simulink model "pendulumss"  (R2021a)
settings: Solver=VariableStepAuto  StartTime=0.0  StopTime=2  RelTol=1e-3
undefined symbols (not defined in the file or in its folder): kC_Z, repC
settings Model: Creator=kaled  LastModifiedBy=kaled

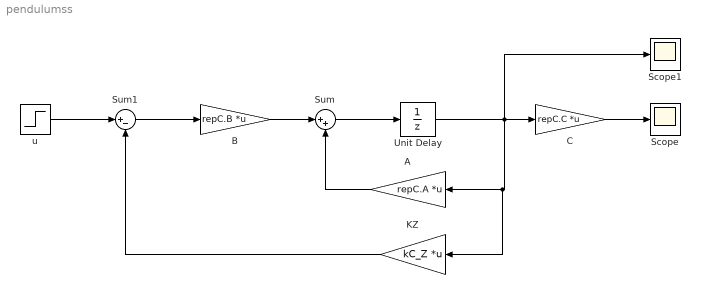
== system pendulumss ==
  A : Gain  Gain=repC.A  Multiplication=Matrix(K*u)
  B : Gain  Gain=repC.B  Multiplication=Matrix(K*u)
  C : Gain  Gain=repC.C  Multiplication=Matrix(K*u)
  KZ : Gain  Gain=kC_Z  Multiplication=Matrix(K*u)
  Scope : Scope
  Scope1 : Scope
  Sum : Sum  Inputs=|++
  Sum1 : Sum  Inputs=|+-
  Unit Delay : UnitDelay  InitialCondition=[0 0.1 pi/6 0]  SampleTime=0.0137  HasFrameUpgradeWarning=on
  u : Step  Time=0  After=0  SampleTime=0
  wires:
  Sum/1 -> Unit Delay/1
  B/1 -> Sum/1
  A/1 -> Sum/2
  Unit Delay/1 -> KZ/1, A/1, Scope1/1, C/1
  C/1 -> Scope/1
  KZ/1 -> Sum1/2
  Sum1/1 -> B/1
  u/1 -> Sum1/1
